simulink model "UNIFIER_dyn3DOF"  (R2023b)
settings: Solver=VariableStepAuto  StartTime=0.0  StopTime=0  RelTol=1e-3
InitFcn:
  | UNIFIER_LOAD
values from neighbouring files (symbols this model uses):
  b = 20.11467    [UNIFIER_LOAD.m]    (also in UNIFIER_LOAD.mat; UNIFIER_LOAD_ROM.m; UNIFIER_LOAD_ROM.mat)
  c = 1.43676    [UNIFIER_LOAD.m]    (also in UNIFIER_LOAD.mat; UNIFIER_LOAD_ROM.m; UNIFIER_LOAD_ROM.mat)
  dp_DEP =     [UNIFIER_LOAD.mat]    (also in UNIFIER_LOAD_ROM.mat)
  dp_FUSE_FIN =     [UNIFIER_LOAD.mat]
  dp_HTU =     [UNIFIER_LOAD.mat]    (also in UNIFIER_LOAD_ROM.mat)
  dp_VTAIL =     [UNIFIER_LOAD.mat]
  dp_VTAIL_INDUCED =     [UNIFIER_LOAD.mat]
  dp_WING_root =     [UNIFIER_LOAD.mat]
  dp_WING_tip =     [UNIFIER_LOAD.mat]
  I = [23600,     -0,  -1740 ... (first row only)    [UNIFIER_LOAD.m]    (also in UNIFIER_LOAD.mat = [23600  0  -1740; 0  89800  0; -1740  0  102000]; UNIFIER_LOAD_ROM.m = [23600,     -0,   -1740; UNIFIER_LOAD_ROM.mat = [23600  0  -1740; 0  89800  0; -1740  0  102000])
  m = 7057    [UNIFIER_LOAD.m]    (also in UNIFIER_LOAD.mat; UNIFIER_LOAD_ROM.m; UNIFIER_LOAD_ROM.mat)
  S = 29.98388    [UNIFIER_LOAD.m]    (also in UNIFIER_LOAD.mat; UNIFIER_LOAD_ROM.m; UNIFIER_LOAD_ROM.mat)
  vtail_nodes = [dp_VTAIL.Xs_LE;     dp_VTAIL.Ys_LE;     dp_VTAIL.Zs_LE]    [UNIFIER_LOAD.m]    (also in UNIFIER_LOAD.mat = [-16.4894695282 -2.83441376686 -2.73765826225 -16.1370849609)
  wing_nodes = [fliplr(dp_WING_tip.LE_Xs),fliplr(dp_WING_root.LE_Xs),dp_WING_root.LE_Xs,dp_WING_tip.LE_Xs;     fliplr(-dp_WING_tip.LE_Ys),fliplr(-dp_WING_root.LE_Ys),dp_WING_root.LE_Ys,dp_WING_tip.LE_Ys;     fliplr(dp_WING_tip.LE_Zs),fliplr(dp_WING_root.LE_Zs),dp_WING_root.LE_Zs,dp_WING_tip.LE_Zs]    [UNIFIER_LOAD.m]    (also in UNIFIER_LOAD.mat = [-7.70795631409 -9.67500019073 -0.98178178072 -7.66801691055)
  xyz_cg = [-8.09,0,-0.2]    [UNIFIER_LOAD.m]    (also in UNIFIER_LOAD.mat = [-8.09 0 -0.2]; UNIFIER_LOAD_ROM.m; UNIFIER_LOAD_ROM.mat = [-8.09 0 -0.2])
  xyz_DEP = [ -6.9629998	-6.9210000	-6.8660002	-6.8099999	-6.7540002	-6.6999998	-6.6999998	-6.7540002	-6.8099999	-6.8660002	-6.9210000	-6.9629998 ... (first row only)    [UNIFIER_LOAD.m]    (also in UNIFIER_LOAD.mat = [-6.9629998 -10.05 -0.90899998 -6.921 -8.4499998 -0.792 -6.8; UNIFIER_LOAD_ROM.m; UNIFIER_LOAD_ROM.mat = [-6.9629998 -10.05 -0.90899998 -6.921 -8.4499998 -0.792 -6.8)
undefined symbols (not defined in the file or in its folder): OBM, unifier_obm
libraries: sharedutil x7, aerolibtransform2 x4, sharedtransform x2, aerolibatmos2 x1, matrix_library x1, shared6dofsys x1, shared6dof x1, simulink x1
(part 2 of 3)

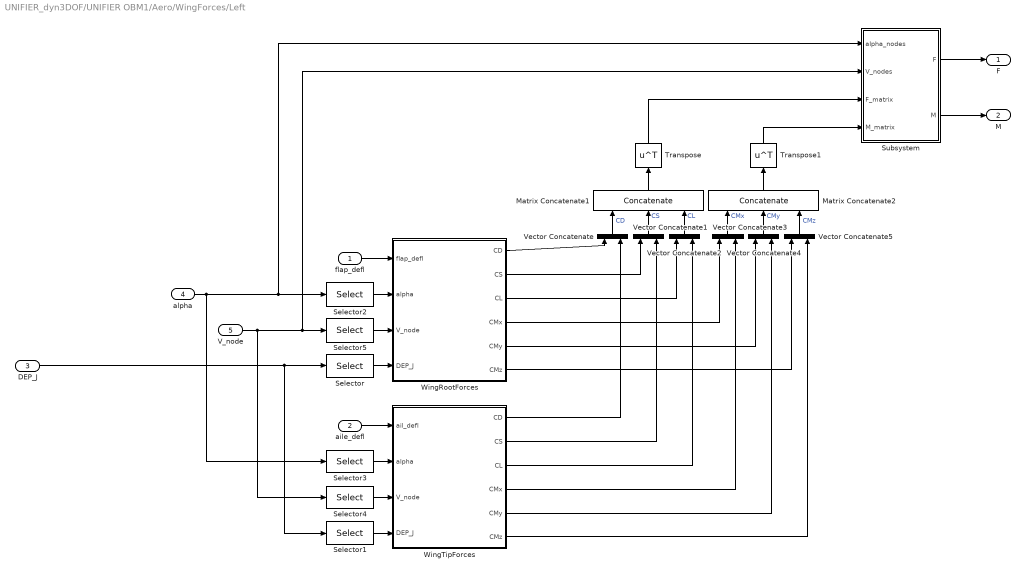
== system UNIFIER_dyn3DOF/UNIFIER OBM1/Aero/WingForces/Left ==
  flap_defl : Inport
  aile_defl : Inport  Port=2
  DEP_J : Inport  Port=3  PortDimensions=6
  alpha : Inport  Port=4  PortDimensions=7
  V_node : Inport  Port=5  PortDimensions=7
  Matrix Concatenate1 : Concatenate  NumInputs=3  Mode=Multidimensional array  ConcatenateDimension=2
  Matrix Concatenate2 : Concatenate  NumInputs=3  Mode=Multidimensional array  ConcatenateDimension=2
  Selector : Selector  InputPortWidth=6  IndexOptions=Index vector (dialog)  Indices=[1,2,3,4,5]  OutputSizes=1
  Selector1 : Selector  InputPortWidth=6  IndexOptions=Index vector (dialog)  Indices=[5,6]  OutputSizes=1
  Selector2 : Selector  InputPortWidth=7  IndexOptions=Index vector (dialog)  Indices=[1,2,3,4,5]  OutputSizes=1
  Selector3 : Selector  InputPortWidth=7  IndexOptions=Index vector (dialog)  Indices=[6,7]  OutputSizes=1
  Selector4 : Selector  InputPortWidth=7  IndexOptions=Index vector (dialog)  Indices=[6,7]  OutputSizes=1
  Selector5 : Selector  InputPortWidth=7  IndexOptions=Index vector (dialog)  Indices=[1,2,3,4,5]  OutputSizes=1
  Subsystem : Subsystem
  Transpose : Math  Operator=transpose
  Transpose1 : Math  Operator=transpose
  Vector Concatenate{,1..5} (6 alike) : Concatenate
  WingRootForces : Subsystem
  WingTipForces : Subsystem
  F : Outport
  M : Outport  Port=2
  wires:
  Subsystem/2(M) -> M/1
  Subsystem/1(F) -> F/1
  Transpose1/1 -> Subsystem/4(M_matrix)
  Transpose/1 -> Subsystem/3(F_matrix)
  Matrix Concatenate2/1 -> Transpose1/1
  Vector Concatenate5/1 -> Matrix Concatenate2/3  "CMz"
  Vector Concatenate4/1 -> Matrix Concatenate2/2  "CMy"
  Vector Concatenate3/1 -> Matrix Concatenate2/1  "CMx"
  Vector Concatenate2/1 -> Matrix Concatenate1/3  "CL"
  Vector Concatenate/1 -> Matrix Concatenate1/1  "CD"
  Matrix Concatenate1/1 -> Transpose/1
  Vector Concatenate1/1 -> Matrix Concatenate1/2  "CS"
  WingRootForces/5(CMy) -> Vector Concatenate4/1
  WingRootForces/4(CMx) -> Vector Concatenate3/1
  WingRootForces/3(CL) -> Vector Concatenate2/1
  WingRootForces/2(CS) -> Vector Concatenate1/1
  Selector5/1 -> WingRootForces/3(V_node)
  Selector4/1 -> WingTipForces/3(V_node)
  Selector3/1 -> WingTipForces/2(alpha)
  Selector2/1 -> WingRootForces/2(alpha)
  aile_defl/1 -> WingTipForces/1(ail_defl)
  WingTipForces/4(CMx) -> Vector Concatenate3/2
  WingTipForces/5(CMy) -> Vector Concatenate4/2
  WingTipForces/3(CL) -> Vector Concatenate2/2
  WingTipForces/2(CS) -> Vector Concatenate1/2
  WingTipForces/6(CMz) -> Vector Concatenate5/2
  WingTipForces/1(CD) -> Vector Concatenate/2
  WingRootForces/6(CMz) -> Vector Concatenate5/1
  Selector1/1 -> WingTipForces/4(DEP_J)
  WingRootForces/1(CD) -> Vector Concatenate/1
  V_node/1 -> Selector5/1, Subsystem/2(V_nodes), Selector4/1
  Selector/1 -> WingRootForces/4(DEP_J)
  DEP_J/1 -> Selector/1, Selector1/1
  alpha/1 -> Selector3/1, Selector2/1, Subsystem/1(alpha_nodes)
  flap_defl/1 -> WingRootForces/1(flap_defl)

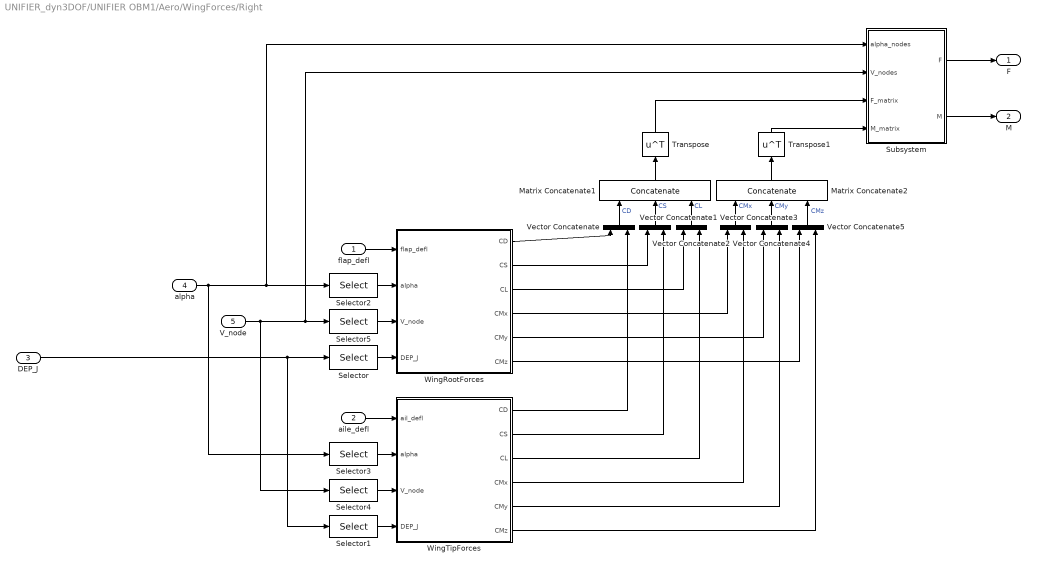
== system UNIFIER_dyn3DOF/UNIFIER OBM1/Aero/WingForces/Right ==
  flap_defl : Inport
  aile_defl : Inport  Port=2
  DEP_J : Inport  Port=3  PortDimensions=6
  alpha : Inport  Port=4  PortDimensions=7
  V_node : Inport  Port=5  PortDimensions=7
  Matrix Concatenate1 : Concatenate  NumInputs=3  Mode=Multidimensional array  ConcatenateDimension=2
  Matrix Concatenate2 : Concatenate  NumInputs=3  Mode=Multidimensional array  ConcatenateDimension=2
  Selector : Selector  InputPortWidth=6  IndexOptions=Index vector (dialog)  Indices=[1,2,3,4,5]  OutputSizes=1
  Selector1 : Selector  InputPortWidth=6  IndexOptions=Index vector (dialog)  Indices=[5,6]  OutputSizes=1
  Selector2 : Selector  InputPortWidth=7  IndexOptions=Index vector (dialog)  Indices=[1,2,3,4,5]  OutputSizes=1
  Selector3 : Selector  InputPortWidth=7  IndexOptions=Index vector (dialog)  Indices=[6,7]  OutputSizes=1
  Selector4 : Selector  InputPortWidth=7  IndexOptions=Index vector (dialog)  Indices=[6,7]  OutputSizes=1
  Selector5 : Selector  InputPortWidth=7  IndexOptions=Index vector (dialog)  Indices=[1,2,3,4,5]  OutputSizes=1
  Subsystem : Subsystem
  Transpose : Math  Operator=transpose
  Transpose1 : Math  Operator=transpose
  Vector Concatenate{,1..5} (6 alike) : Concatenate
  WingRootForces : Subsystem
  WingTipForces : Subsystem
  F : Outport
  M : Outport  Port=2
  wires:
  Subsystem/2(M) -> M/1
  Subsystem/1(F) -> F/1
  Transpose1/1 -> Subsystem/4(M_matrix)
  Transpose/1 -> Subsystem/3(F_matrix)
  Matrix Concatenate2/1 -> Transpose1/1
  Vector Concatenate5/1 -> Matrix Concatenate2/3  "CMz"
  Vector Concatenate4/1 -> Matrix Concatenate2/2  "CMy"
  Vector Concatenate3/1 -> Matrix Concatenate2/1  "CMx"
  Vector Concatenate2/1 -> Matrix Concatenate1/3  "CL"
  Vector Concatenate/1 -> Matrix Concatenate1/1  "CD"
  Matrix Concatenate1/1 -> Transpose/1
  Vector Concatenate1/1 -> Matrix Concatenate1/2  "CS"
  WingRootForces/5(CMy) -> Vector Concatenate4/1
  WingRootForces/4(CMx) -> Vector Concatenate3/1
  WingRootForces/3(CL) -> Vector Concatenate2/1
  WingRootForces/2(CS) -> Vector Concatenate1/1
  Selector5/1 -> WingRootForces/3(V_node)
  Selector4/1 -> WingTipForces/3(V_node)
  Selector3/1 -> WingTipForces/2(alpha)
  Selector2/1 -> WingRootForces/2(alpha)
  aile_defl/1 -> WingTipForces/1(ail_defl)
  WingTipForces/4(CMx) -> Vector Concatenate3/2
  WingTipForces/5(CMy) -> Vector Concatenate4/2
  WingTipForces/3(CL) -> Vector Concatenate2/2
  WingTipForces/2(CS) -> Vector Concatenate1/2
  WingTipForces/6(CMz) -> Vector Concatenate5/2
  WingTipForces/1(CD) -> Vector Concatenate/2
  WingRootForces/6(CMz) -> Vector Concatenate5/1
  Selector1/1 -> WingTipForces/4(DEP_J)
  WingRootForces/1(CD) -> Vector Concatenate/1
  V_node/1 -> Selector5/1, Subsystem/2(V_nodes), Selector4/1
  Selector/1 -> WingRootForces/4(DEP_J)
  DEP_J/1 -> Selector/1, Selector1/1
  alpha/1 -> Selector3/1, Selector2/1, Subsystem/1(alpha_nodes)
  flap_defl/1 -> WingRootForces/1(flap_defl)

== system UNIFIER_dyn3DOF/UNIFIER OBM1/Aero/WingForces/Subsystem ==
  DEP_J : Inport
  alpha_nodes : Inport  Port=2
  V_nodes : Inport  Port=3
  Demux1 : Demux  Outputs=2
  Demux2 : Demux  Outputs=2
  Demux3 : Demux  Outputs=2
  Selector : Selector  InputPortWidth=6  IndexOptions=Index vector (dialog)  Indices=[6,5,4,3,2,1]  OutputSizes=1
  Selector1 : Selector  InputPortWidth=7  IndexOptions=Index vector (dialog)  Indices=[7,6,5,4,3,2,1]  OutputSizes=1
  Selector2 : Selector  InputPortWidth=7  IndexOptions=Index vector (dialog)  Indices=[7,6,5,4,3,2,1]  OutputSizes=1
  DEP_J_Left : Outport  PortDimensions=6
  alpha_nodes_Left : Outport  Port=2  PortDimensions=7
  V_nodes_Left : Outport  Port=3  PortDimensions=7
  DEP_J_Right : Outport  Port=4  PortDimensions=6
  alpha_nodes_Right : Outport  Port=5  PortDimensions=7
  V_nodes_Right : Outport  Port=6  PortDimensions=7
  wires:
  Demux3/2 -> V_nodes_Right/1
  V_nodes/1 -> Demux3/1
  Selector2/1 -> V_nodes_Left/1
  Demux3/1 -> Selector2/1
  Demux1/1 -> Selector1/1
  Demux1/2 -> alpha_nodes_Right/1
  alpha_nodes/1 -> Demux1/1
  Selector1/1 -> alpha_nodes_Left/1
  Selector/1 -> DEP_J_Left/1
  DEP_J/1 -> Demux2/1
  Demux2/1 -> Selector/1
  Demux2/2 -> DEP_J_Right/1

== system UNIFIER_dyn3DOF/UNIFIER OBM1/EOMandEnviroment/EOM/Subsystem ==
  p q r : Inport
  phi theta psi : Inport  Port=2
  Mux1 : Mux  Inputs=[3 3 3]
  Mux2 : Mux  Inputs=3
  phidot : Fcn  Expr=u[1]+(u[2]*u[4]+u[3]*u[7])*(u[5]/u[8])
  psidot : Fcn  Expr=(u[2]*u[4]+u[3]*u[7])/u[8]
  sincos : Trigonometry  Operator=sincos
  thetadot : Fcn  Expr=u[2]*u[7]-u[3]*u[4]
  phidot thetadot psidot : Outport  InitialOutput=0  VectorParamsAs1DForOutWhenUnconnected=off
  wires:
  sincos/2 -> Mux1/3
  phi theta psi/1 -> sincos/1
  phidot/1 -> Mux2/1
  Mux2/1 -> phidot thetadot psidot/1
  p q r/1 -> Mux1/1
  thetadot/1 -> Mux2/2
  psidot/1 -> Mux2/3
  sincos/1 -> Mux1/2
  Mux1/1 -> thetadot/1, phidot/1, psidot/1

== system UNIFIER_dyn3DOF/UNIFIER OBM1/Subsystems/DEP1/AngularVelocityComponent ==
  r : Inport
  Constant : Constant  Value=xyz_DEP
  Constant4 : Constant  Value=xyz_cg
  Gain : Gain  Gain=ones(1,12)
  Product : Product
  Reshape : Reshape
  Reshape3 : Reshape
  Selector1 : Selector  NumberOfDimensions=2  InputPortWidth=6  IndexOptions=Index vector (dialog),Select all  Indices=2,1  OutputSizes=1,1
  Selector3 : Selector  InputPortWidth=3  IndexOptions=Index vector (dialog)  Indices=2  OutputSizes=1
  Sum1 : Sum  Inputs=|+-
  u_induced : Outport
  wires:
  Product/1 -> u_induced/1
  Reshape/1 -> Sum1/2
  Constant/1 -> Selector1/1
  r/1 -> Product/1
  Reshape3/1 -> Sum1/1
  Gain/1 -> Reshape3/1
  Selector3/1 -> Gain/1
  Sum1/1 -> Product/2
  Constant4/1 -> Selector3/1
  Selector1/1 -> Reshape/1

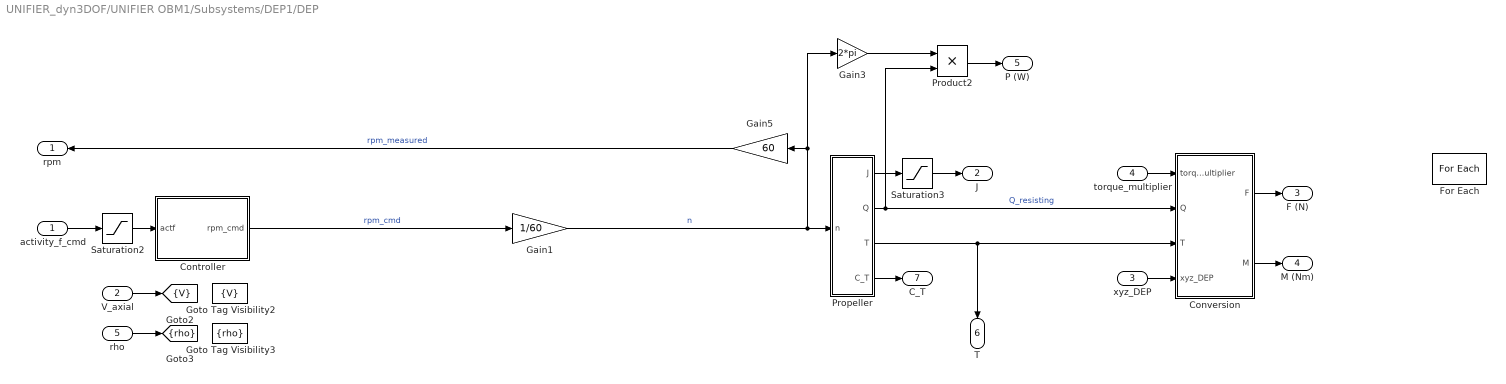
== system UNIFIER_dyn3DOF/UNIFIER OBM1/Subsystems/DEP1/DEP ==
  activity_f_cmd : Inport  Partition=on  PartitionDimension=1  PartitionWidth=1  PartitionOffset=0
  V_axial : Inport  Port=2  Partition=on  PartitionDimension=1  PartitionWidth=1  PartitionOffset=0
  xyz_DEP : Inport  Port=3  Partition=on  PartitionDimension=2  PartitionWidth=1  PartitionOffset=0
  torque_multiplier : Inport  Port=4  Partition=on  PartitionDimension=1  PartitionWidth=1  PartitionOffset=0
  rho : Inport  Port=5
  Controller : Subsystem
  Conversion : Subsystem
  For Each : ForEach  DisableCoverage=on  SpecifiedNumIters=12
  Gain1 : Gain  Gain=1/60
  Gain3 : Gain  Gain=2*pi
  Gain5 : Gain  Gain=60
  Goto Tag Visibility2 : GotoTagVisibility  GotoTag=V
  Goto Tag Visibility3 : GotoTagVisibility  GotoTag=rho
  Product2 : Product
  Propeller : Subsystem
  Saturation2 : Saturate  UpperLimit=1  LowerLimit=0
  Saturation3 : Saturate  UpperLimit=5  LowerLimit=0.2
  rpm : Outport  ConcatenationDimension=1
  J : Outport  Port=2  ConcatenationDimension=1
  F (N) : Outport  Port=3  ConcatenationDimension=2
  M (Nm) : Outport  Port=4  ConcatenationDimension=2
  P (W) : Outport  Port=5  ConcatenationDimension=1
  T : Outport  Port=6  ConcatenationDimension=1
  C_T : Outport  Port=7  ConcatenationDimension=1
  tag scope: V=scoped, rho=scoped
  wires:
  Controller/1(rpm_cmd) -> Gain1/1  "rpm_cmd"
  Saturation2/1 -> Controller/1(actf)
  Propeller/2(Q) -> Conversion/2(Q), Product2/2  "Q_resisting"
  rho/1 -> [rho]
  Propeller/3(T) -> Conversion/3(T), T/1
  Gain5/1 -> rpm/1  "rpm_measured"
  torque_multiplier/1 -> Conversion/1(torque_multiplier)
  Product2/1 -> P (W)/1
  V_axial/1 -> [V]
  Gain1/1 -> Propeller/1(n), Gain5/1, Gain3/1  "n"
  xyz_DEP/1 -> Conversion/4(xyz_DEP)
  Gain3/1 -> Product2/1
  Propeller/1(J) -> Saturation3/1
  activity_f_cmd/1 -> Saturation2/1
  Propeller/4(C_T) -> C_T/1
  Saturation3/1 -> J/1
  Conversion/2(M) -> M (Nm)/1
  Conversion/1(F) -> F (N)/1

== system UNIFIER_dyn3DOF/UNIFIER OBM1/Subsystems/HTU/PropAndMotor ==
  Vrw_mag_eas : Inport
  T_cmd (N) : Inport  Port=2
  1-D Lookup Table : Lookup_n-D  NumberOfTableDimensions=1  BreakpointsForDimension1=dp_HTU.limits.V_low_lim  IndexSearchMethod=Linear search  BeginIndexSearchUsingPreviousIndexResult=on  Table=dp_HTU.limits.T_low_lim  InternalRulePriority=Speed  RndMeth=Simplest
  1-D Lookup Table1 : Lookup_n-D  NumberOfTableDimensions=1  BreakpointsForDimension1=dp_HTU.limits.V_up_lim  IndexSearchMethod=Linear search  BeginIndexSearchUsingPreviousIndexResult=on  Table=dp_HTU.limits.T_up_lim  InternalRulePriority=Speed  RndMeth=Simplest
  P lookup : Lookup_n-D  BreakpointsForDimension1=dp_HTU.V_vec  BreakpointsForDimension2=dp_HTU.T_vec  IndexSearchMethod=Linear search  BeginIndexSearchUsingPreviousIndexResult=on  Table=dp_HTU.P_grid  InternalRulePriority=Speed  RndMeth=Simplest
      settings: InputPortMap=u0,u1
  Saturation Dynamic : simulink/Discontinuities/Saturation Dynamic  OutMin=[]  OutMax=[]  OutDataTypeStr=Inherit: Same as second input  OutDataType=fixdt(1, 16)  OutScaling=2^-10  DoSatur=off
  P (kW) : Outport
  T (N) : Outport  Port=2
  wires:
  Saturation Dynamic/1 -> P lookup/2, T (N)/1
  T_cmd (N)/1 -> Saturation Dynamic/2
  1-D Lookup Table/1 -> Saturation Dynamic/3
  1-D Lookup Table1/1 -> Saturation Dynamic/1
  P lookup/1 -> P (kW)/1
  Vrw_mag_eas/1 -> 1-D Lookup Table1/1, 1-D Lookup Table/1, P lookup/1

== system UNIFIER_dyn3DOF/UNIFIER OBM1/Aero/FinFuselageForces/Subsystem1/Subsystem ==
  beta : Inport
  alpha : Inport  Port=2
  Prelookup : PreLookup  BreakpointsData=dp_FUSE_FIN.beta  IndexSearchMethod=Linear search  BeginIndexSearchUsingPreviousIndexResult=on  ExtrapMethod=Linear
  Prelookup1 : PreLookup  BreakpointsData=dp_FUSE_FIN.aoa  IndexSearchMethod=Linear search  BeginIndexSearchUsingPreviousIndexResult=on  ExtrapMethod=Linear
  Out1 : Outport
  Out2 : Outport  Port=2
  Out3 : Outport  Port=3
  Out4 : Outport  Port=4
  wires:
  Prelookup/2 -> Out2/1
  Prelookup1/2 -> Out4/1
  Prelookup1/1 -> Out3/1
  beta/1 -> Prelookup/1
  alpha/1 -> Prelookup1/1
  Prelookup/1 -> Out1/1

== system UNIFIER_dyn3DOF/UNIFIER OBM1/Aero/VtailForces/Subsystem/CrossProduct1 ==
  r : Inport  Partition=on  PartitionDimension=2  PartitionWidth=1  PartitionOffset=0
  F : Inport  Port=2  Partition=on  PartitionDimension=2  PartitionWidth=1  PartitionOffset=0
  3x3 Cross Product : sharedutil/3x3 Cross Product  aMode=aMode
  CG : Constant  Value=xyz_cg
  Cast : DataTypeConversion  OutDataTypeStr=single  SaturateOnIntegerOverflow=off  RndMeth=Floor
  For Each : ForEach  DisableCoverage=on  SpecifiedNumIters=16
  Minus : Sum  Inputs=+-
  M : Outport  ConcatenationDimension=2
  wires:
  Cast/1 -> Minus/2
  Minus/1 -> 3x3 Cross Product/1
  CG/1 -> Cast/1
  3x3 Cross Product/1 -> M/1
  r/1 -> Minus/1
  F/1 -> 3x3 Cross Product/2

== system UNIFIER_dyn3DOF/UNIFIER OBM1/Aero/VtailForces/VtailForces/WingRootPreLookup ==
  rude_defl_nodes : Inport
  alpha_nodes : Inport  Port=2
  beta_nodes : Inport  Port=3
  Constant8 : Constant  Value=0:15
  Prelookup : PreLookup  BreakpointsData=dp_VTAIL.rude_defl  IndexSearchMethod=Linear search  BeginIndexSearchUsingPreviousIndexResult=on  ExtrapMethod=Linear
  Prelookup1 : PreLookup  BreakpointsData=dp_VTAIL.alphas  IndexSearchMethod=Linear search  BeginIndexSearchUsingPreviousIndexResult=on  ExtrapMethod=Linear
  Prelookup2 : PreLookup  BreakpointsData=dp_VTAIL.betas  IndexSearchMethod=Linear search  BeginIndexSearchUsingPreviousIndexResult=on  ExtrapMethod=Linear
  Out1 : Outport
  Out2 : Outport  Port=2
  Out3 : Outport  Port=3
  Out4 : Outport  Port=4
  Out6 : Outport  Port=5
  Out7 : Outport  Port=6
  Out5 : Outport  Port=7
  wires:
  Prelookup2/2 -> Out7/1
  Prelookup2/1 -> Out6/1
  beta_nodes/1 -> Prelookup2/1
  rude_defl_nodes/1 -> Prelookup/1
  Prelookup1/1 -> Out3/1
  alpha_nodes/1 -> Prelookup1/1
  Prelookup/2 -> Out2/1
  Prelookup1/2 -> Out4/1
  Constant8/1 -> Out5/1
  Prelookup/1 -> Out1/1

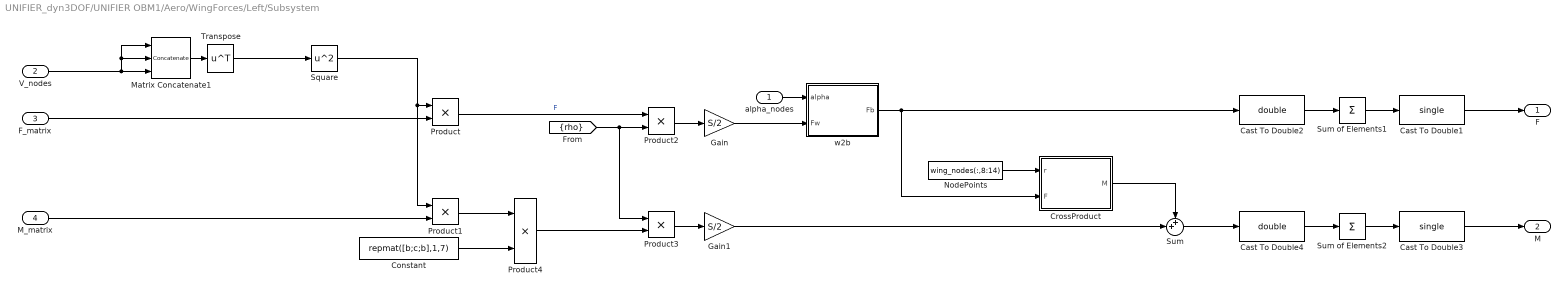
== system UNIFIER_dyn3DOF/UNIFIER OBM1/Aero/WingForces/Left/Subsystem ==
  alpha_nodes : Inport
  V_nodes : Inport  Port=2
  F_matrix : Inport  Port=3
  M_matrix : Inport  Port=4
  Cast To Double1 : DataTypeConversion  OutDataTypeStr=single  SaturateOnIntegerOverflow=off  RndMeth=Floor
  Cast To Double2 : DataTypeConversion  OutDataTypeStr=double  SaturateOnIntegerOverflow=off  RndMeth=Floor
  Cast To Double3 : DataTypeConversion  OutDataTypeStr=single  SaturateOnIntegerOverflow=off  RndMeth=Floor
  Cast To Double4 : DataTypeConversion  OutDataTypeStr=double  SaturateOnIntegerOverflow=off  RndMeth=Floor
  Constant : Constant  Value=repmat([b;c;b],1,7)
  CrossProduct : Subsystem  TreatAsAtomicUnit=on
  Gain : Gain  Gain=S/2
  Gain1 : Gain  Gain=S/2
  Matrix Concatenate1 : Concatenate  NumInputs=3  Mode=Multidimensional array  ConcatenateDimension=2
  NodePoints : Constant  Value=wing_nodes(:,8:14)
  Product{,1..4} (5 alike) : Product
  Square : Math  Operator=square
  Sum : Sum  Inputs=++|
  Sum of Elements1 : Sum  Inputs=+  CollapseMode=Specified dimension  CollapseDim=2
  Sum of Elements2 : Sum  Inputs=+  CollapseMode=Specified dimension  CollapseDim=2
  Transpose : Math  Operator=transpose
  w2b : Subsystem  TreatAsAtomicUnit=on
  F : Outport
  M : Outport  Port=2
  wires:
  Cast To Double3/1 -> M/1
  Sum/1 -> Cast To Double4/1
  Cast To Double4/1 -> Sum of Elements2/1
  Sum of Elements2/1 -> Cast To Double3/1
  Sum of Elements1/1 -> Cast To Double1/1
  Cast To Double2/1 -> Sum of Elements1/1
  alpha_nodes/1 -> w2b/1(alpha)
  Gain/1 -> w2b/2(Fw)
  Cast To Double1/1 -> F/1
  CrossProduct/1(M) -> Sum/1
  NodePoints/1 -> CrossProduct/1(r)
  w2b/1(Fb) -> CrossProduct/2(F), Cast To Double2/1
  Square/1 -> Product/1, Product1/1
  Matrix Concatenate1/1 -> Transpose/1
  Transpose/1 -> Square/1
  V_nodes/1 -> Matrix Concatenate1/3, Matrix Concatenate1/2, Matrix Concatenate1/1
  Product/1 -> Product2/1  "F"
  Gain1/1 -> Sum/2
  Product1/1 -> Product4/1
  M_matrix/1 -> Product1/2
  Product4/1 -> Product3/2
  Constant/1 -> Product4/2
  Product3/1 -> Gain1/1
  [rho] -> Product2/2, Product3/1
  F_matrix/1 -> Product/2
  Product2/1 -> Gain/1

== system UNIFIER_dyn3DOF/UNIFIER OBM1/Aero/WingForces/Left/WingRootForces ==
  flap_defl : Inport
  alpha : Inport  Port=2
  V_node : Inport  Port=3
  DEP_J : Inport  Port=4
  Interpolation Using Prelookup1 : Interpolation_n-D  NumberOfTableDimensions=5  Table=dp_WING_root.CD  ExtrapMethod=Clip  ValidIndexMayReachLast=on  NumSelectionDims=1  InternalRulePriority=Speed  TableDataTypeStr=Inherit: Inherit from 'Table data'
      settings: InputPortMap=u0,u1,u2,u3,u4,u5,u6,u7,u8
  Interpolation Using Prelookup2 : Interpolation_n-D  NumberOfTableDimensions=5  Table=dp_WING_root.CS  ExtrapMethod=Clip  ValidIndexMayReachLast=on  NumSelectionDims=1  InternalRulePriority=Speed  TableDataTypeStr=Inherit: Inherit from 'Table data'
      settings: InputPortMap=u0,u1,u2,u3,u4,u5,u6,u7,u8
  Interpolation Using Prelookup3 : Interpolation_n-D  NumberOfTableDimensions=5  Table=dp_WING_root.CL  ExtrapMethod=Clip  ValidIndexMayReachLast=on  NumSelectionDims=1  InternalRulePriority=Speed  TableDataTypeStr=Inherit: Inherit from 'Table data'
      settings: InputPortMap=u0,u1,u2,u3,u4,u5,u6,u7,u8
  Interpolation Using Prelookup4 : Interpolation_n-D  NumberOfTableDimensions=5  Table=dp_WING_root.CMx  ExtrapMethod=Clip  ValidIndexMayReachLast=on  NumSelectionDims=1  InternalRulePriority=Speed  TableDataTypeStr=Inherit: Inherit from 'Table data'
      settings: InputPortMap=u0,u1,u2,u3,u4,u5,u6,u7,u8
  Interpolation Using Prelookup5 : Interpolation_n-D  NumberOfTableDimensions=5  Table=dp_WING_root.CMy  ExtrapMethod=Clip  ValidIndexMayReachLast=on  NumSelectionDims=1  InternalRulePriority=Speed  TableDataTypeStr=Inherit: Inherit from 'Table data'
      settings: InputPortMap=u0,u1,u2,u3,u4,u5,u6,u7,u8
  Interpolation Using Prelookup6 : Interpolation_n-D  NumberOfTableDimensions=5  Table=dp_WING_root.CMz  ExtrapMethod=Clip  ValidIndexMayReachLast=on  NumSelectionDims=1  InternalRulePriority=Speed  TableDataTypeStr=Inherit: Inherit from 'Table data'
      settings: InputPortMap=u0,u1,u2,u3,u4,u5,u6,u7,u8
  WingRootPreLookup : Subsystem
  CD : Outport
  CS : Outport  Port=2
  CL : Outport  Port=3
  CMx : Outport  Port=4
  CMy : Outport  Port=5
  CMz : Outport  Port=6
  wires:
  Interpolation Using Prelookup6/1 -> CMz/1
  Interpolation Using Prelookup5/1 -> CMy/1
  Interpolation Using Prelookup4/1 -> CMx/1
  Interpolation Using Prelookup3/1 -> CL/1
  Interpolation Using Prelookup2/1 -> CS/1
  alpha/1 -> WingRootPreLookup/2(alpha)
  V_node/1 -> WingRootPreLookup/3(V_node)
  DEP_J/1 -> WingRootPreLookup/4(DEP_J)
  WingRootPreLookup/2(Out2) -> Interpolation Using Prelookup1/2, Interpolation Using Prelookup2/2, Interpolation Using Prelookup3/2, Interpolation Using Prelookup4/2, Interpolation Using Prelookup5/2, Interpolation Using Prelookup6/2
  WingRootPreLookup/6(Out7) -> Interpolation Using Prelookup1/6, Interpolation Using Prelookup2/6, Interpolation Using Prelookup3/6, Interpolation Using Prelookup4/6, Interpolation Using Prelookup5/6, Interpolation Using Prelookup6/6
  Interpolation Using Prelookup1/1 -> CD/1
  WingRootPreLookup/5(Out6) -> Interpolation Using Prelookup2/5, Interpolation Using Prelookup3/5, Interpolation Using Prelookup4/5, Interpolation Using Prelookup5/5, Interpolation Using Prelookup6/5, Interpolation Using Prelookup1/5
  WingRootPreLookup/4(Out4) -> Interpolation Using Prelookup1/4, Interpolation Using Prelookup2/4, Interpolation Using Prelookup3/4, Interpolation Using Prelookup4/4, Interpolation Using Prelookup5/4, Interpolation Using Prelookup6/4
  flap_defl/1 -> WingRootPreLookup/1(flap_defl)
  WingRootPreLookup/7(Out8) -> Interpolation Using Prelookup2/7, Interpolation Using Prelookup3/7, Interpolation Using Prelookup4/7, Interpolation Using Prelookup6/7, Interpolation Using Prelookup5/7, Interpolation Using Prelookup1/7
  WingRootPreLookup/1(Out1) -> Interpolation Using Prelookup1/1, Interpolation Using Prelookup2/1, Interpolation Using Prelookup3/1, Interpolation Using Prelookup4/1, Interpolation Using Prelookup5/1, Interpolation Using Prelookup6/1
  WingRootPreLookup/8(Out9) -> Interpolation Using Prelookup1/8, Interpolation Using Prelookup2/8, Interpolation Using Prelookup3/8, Interpolation Using Prelookup4/8, Interpolation Using Prelookup5/8, Interpolation Using Prelookup6/8
  WingRootPreLookup/3(Out3) -> Interpolation Using Prelookup1/3, Interpolation Using Prelookup2/3, Interpolation Using Prelookup3/3, Interpolation Using Prelookup4/3, Interpolation Using Prelookup5/3, Interpolation Using Prelookup6/3
  WingRootPreLookup/9(Out5) -> Interpolation Using Prelookup1/9, Interpolation Using Prelookup2/9, Interpolation Using Prelookup3/9, Interpolation Using Prelookup4/9, Interpolation Using Prelookup5/9, Interpolation Using Prelookup6/9

== system UNIFIER_dyn3DOF/UNIFIER OBM1/Aero/WingForces/Left/WingTipForces ==
  ail_defl : Inport
  alpha : Inport  Port=2
  V_node : Inport  Port=3
  DEP_J : Inport  Port=4
  Interpolation Using Prelookup1 : Interpolation_n-D  NumberOfTableDimensions=5  Table=dp_WING_tip.CD  ExtrapMethod=Clip  ValidIndexMayReachLast=on  NumSelectionDims=1  InternalRulePriority=Speed  TableDataTypeStr=Inherit: Inherit from 'Table data'
      settings: InputPortMap=u0,u1,u2,u3,u4,u5,u6,u7,u8
  Interpolation Using Prelookup2 : Interpolation_n-D  NumberOfTableDimensions=5  Table=dp_WING_tip.CS  ExtrapMethod=Clip  ValidIndexMayReachLast=on  NumSelectionDims=1  InternalRulePriority=Speed  TableDataTypeStr=Inherit: Inherit from 'Table data'
      settings: InputPortMap=u0,u1,u2,u3,u4,u5,u6,u7,u8
  Interpolation Using Prelookup3 : Interpolation_n-D  NumberOfTableDimensions=5  Table=dp_WING_tip.CL  ExtrapMethod=Clip  ValidIndexMayReachLast=on  NumSelectionDims=1  InternalRulePriority=Speed  TableDataTypeStr=Inherit: Inherit from 'Table data'
      settings: InputPortMap=u0,u1,u2,u3,u4,u5,u6,u7,u8
  Interpolation Using Prelookup4 : Interpolation_n-D  NumberOfTableDimensions=5  Table=dp_WING_tip.CMx  ExtrapMethod=Clip  ValidIndexMayReachLast=on  NumSelectionDims=1  InternalRulePriority=Speed  TableDataTypeStr=Inherit: Inherit from 'Table data'
      settings: InputPortMap=u0,u1,u2,u3,u4,u5,u6,u7,u8
  Interpolation Using Prelookup5 : Interpolation_n-D  NumberOfTableDimensions=5  Table=dp_WING_tip.CMy  ExtrapMethod=Clip  ValidIndexMayReachLast=on  NumSelectionDims=1  InternalRulePriority=Speed  TableDataTypeStr=Inherit: Inherit from 'Table data'
      settings: InputPortMap=u0,u1,u2,u3,u4,u5,u6,u7,u8
  Interpolation Using Prelookup6 : Interpolation_n-D  NumberOfTableDimensions=5  Table=dp_WING_tip.CMz  ExtrapMethod=Clip  ValidIndexMayReachLast=on  NumSelectionDims=1  InternalRulePriority=Speed  TableDataTypeStr=Inherit: Inherit from 'Table data'
      settings: InputPortMap=u0,u1,u2,u3,u4,u5,u6,u7,u8
  WingRootPreLookup : Subsystem
  CD : Outport
  CS : Outport  Port=2
  CL : Outport  Port=3
  CMx : Outport  Port=4
  CMy : Outport  Port=5
  CMz : Outport  Port=6
  wires:
  Interpolation Using Prelookup6/1 -> CMz/1
  Interpolation Using Prelookup5/1 -> CMy/1
  Interpolation Using Prelookup4/1 -> CMx/1
  Interpolation Using Prelookup3/1 -> CL/1
  Interpolation Using Prelookup2/1 -> CS/1
  alpha/1 -> WingRootPreLookup/2(alpha)
  V_node/1 -> WingRootPreLookup/3(V_node)
  DEP_J/1 -> WingRootPreLookup/4(DEP_J)
  WingRootPreLookup/2(Out2) -> Interpolation Using Prelookup1/2, Interpolation Using Prelookup2/2, Interpolation Using Prelookup3/2, Interpolation Using Prelookup4/2, Interpolation Using Prelookup5/2, Interpolation Using Prelookup6/2
  WingRootPreLookup/6(Out7) -> Interpolation Using Prelookup1/6, Interpolation Using Prelookup2/6, Interpolation Using Prelookup3/6, Interpolation Using Prelookup4/6, Interpolation Using Prelookup5/6, Interpolation Using Prelookup6/6
  Interpolation Using Prelookup1/1 -> CD/1
  WingRootPreLookup/5(Out6) -> Interpolation Using Prelookup2/5, Interpolation Using Prelookup3/5, Interpolation Using Prelookup4/5, Interpolation Using Prelookup5/5, Interpolation Using Prelookup6/5, Interpolation Using Prelookup1/5
  WingRootPreLookup/4(Out4) -> Interpolation Using Prelookup1/4, Interpolation Using Prelookup2/4, Interpolation Using Prelookup3/4, Interpolation Using Prelookup4/4, Interpolation Using Prelookup5/4, Interpolation Using Prelookup6/4
  ail_defl/1 -> WingRootPreLookup/1(ail_defl)
  WingRootPreLookup/7(Out8) -> Interpolation Using Prelookup1/7, Interpolation Using Prelookup2/7, Interpolation Using Prelookup3/7, Interpolation Using Prelookup4/7, Interpolation Using Prelookup6/7, Interpolation Using Prelookup5/7
  WingRootPreLookup/1(Out1) -> Interpolation Using Prelookup1/1, Interpolation Using Prelookup2/1, Interpolation Using Prelookup3/1, Interpolation Using Prelookup4/1, Interpolation Using Prelookup5/1, Interpolation Using Prelookup6/1
  WingRootPreLookup/8(Out9) -> Interpolation Using Prelookup1/8, Interpolation Using Prelookup2/8, Interpolation Using Prelookup3/8, Interpolation Using Prelookup4/8, Interpolation Using Prelookup5/8, Interpolation Using Prelookup6/8
  WingRootPreLookup/3(Out3) -> Interpolation Using Prelookup1/3, Interpolation Using Prelookup2/3, Interpolation Using Prelookup3/3, Interpolation Using Prelookup4/3, Interpolation Using Prelookup5/3, Interpolation Using Prelookup6/3
  WingRootPreLookup/9(Out5) -> Interpolation Using Prelookup1/9, Interpolation Using Prelookup2/9, Interpolation Using Prelookup3/9, Interpolation Using Prelookup4/9, Interpolation Using Prelookup5/9, Interpolation Using Prelookup6/9

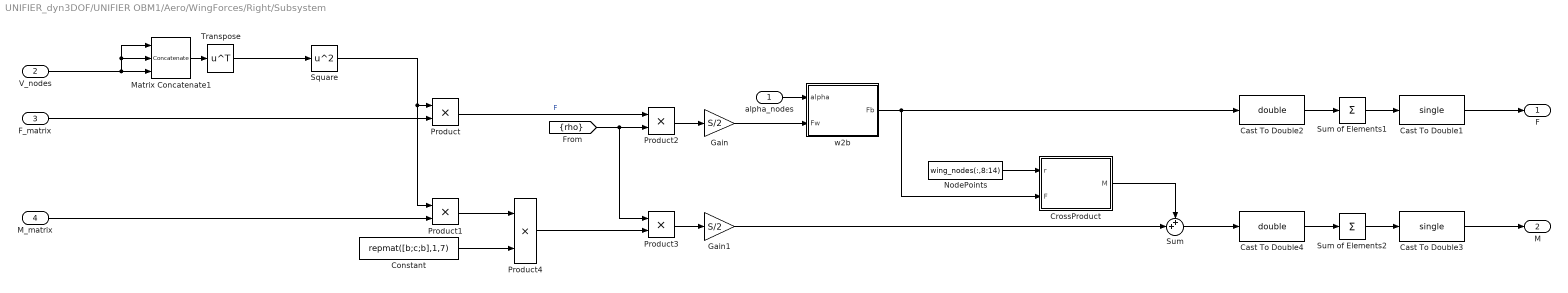
== system UNIFIER_dyn3DOF/UNIFIER OBM1/Aero/WingForces/Right/Subsystem ==
  alpha_nodes : Inport
  V_nodes : Inport  Port=2
  F_matrix : Inport  Port=3
  M_matrix : Inport  Port=4
  Cast To Double1 : DataTypeConversion  OutDataTypeStr=single  SaturateOnIntegerOverflow=off  RndMeth=Floor
  Cast To Double2 : DataTypeConversion  OutDataTypeStr=double  SaturateOnIntegerOverflow=off  RndMeth=Floor
  Cast To Double3 : DataTypeConversion  OutDataTypeStr=single  SaturateOnIntegerOverflow=off  RndMeth=Floor
  Cast To Double4 : DataTypeConversion  OutDataTypeStr=double  SaturateOnIntegerOverflow=off  RndMeth=Floor
  Constant : Constant  Value=repmat([b;c;b],1,7)
  CrossProduct : Subsystem  TreatAsAtomicUnit=on
  Gain : Gain  Gain=S/2
  Gain1 : Gain  Gain=S/2
  Matrix Concatenate1 : Concatenate  NumInputs=3  Mode=Multidimensional array  ConcatenateDimension=2
  NodePoints : Constant  Value=wing_nodes(:,8:14)
  Product{,1..4} (5 alike) : Product
  Square : Math  Operator=square
  Sum : Sum  Inputs=++|
  Sum of Elements1 : Sum  Inputs=+  CollapseMode=Specified dimension  CollapseDim=2
  Sum of Elements2 : Sum  Inputs=+  CollapseMode=Specified dimension  CollapseDim=2
  Transpose : Math  Operator=transpose
  w2b : Subsystem  TreatAsAtomicUnit=on
  F : Outport
  M : Outport  Port=2
  wires:
  Cast To Double3/1 -> M/1
  Sum/1 -> Cast To Double4/1
  Cast To Double4/1 -> Sum of Elements2/1
  Sum of Elements2/1 -> Cast To Double3/1
  Sum of Elements1/1 -> Cast To Double1/1
  Cast To Double2/1 -> Sum of Elements1/1
  alpha_nodes/1 -> w2b/1(alpha)
  Gain/1 -> w2b/2(Fw)
  Cast To Double1/1 -> F/1
  CrossProduct/1(M) -> Sum/1
  NodePoints/1 -> CrossProduct/1(r)
  w2b/1(Fb) -> CrossProduct/2(F), Cast To Double2/1
  Square/1 -> Product/1, Product1/1
  Matrix Concatenate1/1 -> Transpose/1
  Transpose/1 -> Square/1
  V_nodes/1 -> Matrix Concatenate1/3, Matrix Concatenate1/2, Matrix Concatenate1/1
  Product/1 -> Product2/1  "F"
  Gain1/1 -> Sum/2
  Product1/1 -> Product4/1
  M_matrix/1 -> Product1/2
  Product4/1 -> Product3/2
  Constant/1 -> Product4/2
  Product3/1 -> Gain1/1
  [rho] -> Product2/2, Product3/1
  F_matrix/1 -> Product/2
  Product2/1 -> Gain/1

== system UNIFIER_dyn3DOF/UNIFIER OBM1/Aero/WingForces/Right/WingRootForces ==
  flap_defl : Inport
  alpha : Inport  Port=2
  V_node : Inport  Port=3
  DEP_J : Inport  Port=4
  Interpolation Using Prelookup1 : Interpolation_n-D  NumberOfTableDimensions=5  Table=dp_WING_root.CD  ExtrapMethod=Clip  ValidIndexMayReachLast=on  NumSelectionDims=1  InternalRulePriority=Speed  TableDataTypeStr=Inherit: Inherit from 'Table data'
      settings: InputPortMap=u0,u1,u2,u3,u4,u5,u6,u7,u8
  Interpolation Using Prelookup2 : Interpolation_n-D  NumberOfTableDimensions=5  Table=dp_WING_root.CS  ExtrapMethod=Clip  ValidIndexMayReachLast=on  NumSelectionDims=1  InternalRulePriority=Speed  TableDataTypeStr=Inherit: Inherit from 'Table data'
      settings: InputPortMap=u0,u1,u2,u3,u4,u5,u6,u7,u8
  Interpolation Using Prelookup3 : Interpolation_n-D  NumberOfTableDimensions=5  Table=dp_WING_root.CL  ExtrapMethod=Clip  ValidIndexMayReachLast=on  NumSelectionDims=1  InternalRulePriority=Speed  TableDataTypeStr=Inherit: Inherit from 'Table data'
      settings: InputPortMap=u0,u1,u2,u3,u4,u5,u6,u7,u8
  Interpolation Using Prelookup4 : Interpolation_n-D  NumberOfTableDimensions=5  Table=dp_WING_root.CMx  ExtrapMethod=Clip  ValidIndexMayReachLast=on  NumSelectionDims=1  InternalRulePriority=Speed  TableDataTypeStr=Inherit: Inherit from 'Table data'
      settings: InputPortMap=u0,u1,u2,u3,u4,u5,u6,u7,u8
  Interpolation Using Prelookup5 : Interpolation_n-D  NumberOfTableDimensions=5  Table=dp_WING_root.CMy  ExtrapMethod=Clip  ValidIndexMayReachLast=on  NumSelectionDims=1  InternalRulePriority=Speed  TableDataTypeStr=Inherit: Inherit from 'Table data'
      settings: InputPortMap=u0,u1,u2,u3,u4,u5,u6,u7,u8
  Interpolation Using Prelookup6 : Interpolation_n-D  NumberOfTableDimensions=5  Table=dp_WING_root.CMz  ExtrapMethod=Clip  ValidIndexMayReachLast=on  NumSelectionDims=1  InternalRulePriority=Speed  TableDataTypeStr=Inherit: Inherit from 'Table data'
      settings: InputPortMap=u0,u1,u2,u3,u4,u5,u6,u7,u8
  WingRootPreLookup : Subsystem
  CD : Outport
  CS : Outport  Port=2
  CL : Outport  Port=3
  CMx : Outport  Port=4
  CMy : Outport  Port=5
  CMz : Outport  Port=6
  wires:
  Interpolation Using Prelookup6/1 -> CMz/1
  Interpolation Using Prelookup5/1 -> CMy/1
  Interpolation Using Prelookup4/1 -> CMx/1
  Interpolation Using Prelookup3/1 -> CL/1
  Interpolation Using Prelookup2/1 -> CS/1
  alpha/1 -> WingRootPreLookup/2(alpha)
  V_node/1 -> WingRootPreLookup/3(V_node)
  DEP_J/1 -> WingRootPreLookup/4(DEP_J)
  WingRootPreLookup/2(Out2) -> Interpolation Using Prelookup1/2, Interpolation Using Prelookup2/2, Interpolation Using Prelookup3/2, Interpolation Using Prelookup4/2, Interpolation Using Prelookup5/2, Interpolation Using Prelookup6/2
  WingRootPreLookup/6(Out7) -> Interpolation Using Prelookup1/6, Interpolation Using Prelookup2/6, Interpolation Using Prelookup3/6, Interpolation Using Prelookup4/6, Interpolation Using Prelookup5/6, Interpolation Using Prelookup6/6
  Interpolation Using Prelookup1/1 -> CD/1
  WingRootPreLookup/5(Out6) -> Interpolation Using Prelookup2/5, Interpolation Using Prelookup3/5, Interpolation Using Prelookup4/5, Interpolation Using Prelookup5/5, Interpolation Using Prelookup6/5, Interpolation Using Prelookup1/5
  WingRootPreLookup/4(Out4) -> Interpolation Using Prelookup1/4, Interpolation Using Prelookup2/4, Interpolation Using Prelookup3/4, Interpolation Using Prelookup4/4, Interpolation Using Prelookup5/4, Interpolation Using Prelookup6/4
  flap_defl/1 -> WingRootPreLookup/1(flap_defl)
  WingRootPreLookup/7(Out8) -> Interpolation Using Prelookup2/7, Interpolation Using Prelookup3/7, Interpolation Using Prelookup4/7, Interpolation Using Prelookup6/7, Interpolation Using Prelookup5/7, Interpolation Using Prelookup1/7
  WingRootPreLookup/1(Out1) -> Interpolation Using Prelookup1/1, Interpolation Using Prelookup2/1, Interpolation Using Prelookup3/1, Interpolation Using Prelookup4/1, Interpolation Using Prelookup5/1, Interpolation Using Prelookup6/1
  WingRootPreLookup/8(Out9) -> Interpolation Using Prelookup1/8, Interpolation Using Prelookup2/8, Interpolation Using Prelookup3/8, Interpolation Using Prelookup4/8, Interpolation Using Prelookup5/8, Interpolation Using Prelookup6/8
  WingRootPreLookup/3(Out3) -> Interpolation Using Prelookup1/3, Interpolation Using Prelookup2/3, Interpolation Using Prelookup3/3, Interpolation Using Prelookup4/3, Interpolation Using Prelookup5/3, Interpolation Using Prelookup6/3
  WingRootPreLookup/9(Out5) -> Interpolation Using Prelookup1/9, Interpolation Using Prelookup2/9, Interpolation Using Prelookup3/9, Interpolation Using Prelookup4/9, Interpolation Using Prelookup5/9, Interpolation Using Prelookup6/9

== system UNIFIER_dyn3DOF/UNIFIER OBM1/Aero/WingForces/Right/WingTipForces ==
  ail_defl : Inport
  alpha : Inport  Port=2
  V_node : Inport  Port=3
  DEP_J : Inport  Port=4
  Interpolation Using Prelookup1 : Interpolation_n-D  NumberOfTableDimensions=5  Table=dp_WING_tip.CD  ExtrapMethod=Clip  ValidIndexMayReachLast=on  NumSelectionDims=1  InternalRulePriority=Speed  TableDataTypeStr=Inherit: Inherit from 'Table data'
      settings: InputPortMap=u0,u1,u2,u3,u4,u5,u6,u7,u8
  Interpolation Using Prelookup2 : Interpolation_n-D  NumberOfTableDimensions=5  Table=dp_WING_tip.CS  ExtrapMethod=Clip  ValidIndexMayReachLast=on  NumSelectionDims=1  InternalRulePriority=Speed  TableDataTypeStr=Inherit: Inherit from 'Table data'
      settings: InputPortMap=u0,u1,u2,u3,u4,u5,u6,u7,u8
  Interpolation Using Prelookup3 : Interpolation_n-D  NumberOfTableDimensions=5  Table=dp_WING_tip.CL  ExtrapMethod=Clip  ValidIndexMayReachLast=on  NumSelectionDims=1  InternalRulePriority=Speed  TableDataTypeStr=Inherit: Inherit from 'Table data'
      settings: InputPortMap=u0,u1,u2,u3,u4,u5,u6,u7,u8
  Interpolation Using Prelookup4 : Interpolation_n-D  NumberOfTableDimensions=5  Table=dp_WING_tip.CMx  ExtrapMethod=Clip  ValidIndexMayReachLast=on  NumSelectionDims=1  InternalRulePriority=Speed  TableDataTypeStr=Inherit: Inherit from 'Table data'
      settings: InputPortMap=u0,u1,u2,u3,u4,u5,u6,u7,u8
  Interpolation Using Prelookup5 : Interpolation_n-D  NumberOfTableDimensions=5  Table=dp_WING_tip.CMy  ExtrapMethod=Clip  ValidIndexMayReachLast=on  NumSelectionDims=1  InternalRulePriority=Speed  TableDataTypeStr=Inherit: Inherit from 'Table data'
      settings: InputPortMap=u0,u1,u2,u3,u4,u5,u6,u7,u8
  Interpolation Using Prelookup6 : Interpolation_n-D  NumberOfTableDimensions=5  Table=dp_WING_tip.CMz  ExtrapMethod=Clip  ValidIndexMayReachLast=on  NumSelectionDims=1  InternalRulePriority=Speed  TableDataTypeStr=Inherit: Inherit from 'Table data'
      settings: InputPortMap=u0,u1,u2,u3,u4,u5,u6,u7,u8
  WingRootPreLookup : Subsystem
  CD : Outport
  CS : Outport  Port=2
  CL : Outport  Port=3
  CMx : Outport  Port=4
  CMy : Outport  Port=5
  CMz : Outport  Port=6
  wires:
  Interpolation Using Prelookup6/1 -> CMz/1
  Interpolation Using Prelookup5/1 -> CMy/1
  Interpolation Using Prelookup4/1 -> CMx/1
  Interpolation Using Prelookup3/1 -> CL/1
  Interpolation Using Prelookup2/1 -> CS/1
  alpha/1 -> WingRootPreLookup/2(alpha)
  V_node/1 -> WingRootPreLookup/3(V_node)
  DEP_J/1 -> WingRootPreLookup/4(DEP_J)
  WingRootPreLookup/2(Out2) -> Interpolation Using Prelookup1/2, Interpolation Using Prelookup2/2, Interpolation Using Prelookup3/2, Interpolation Using Prelookup4/2, Interpolation Using Prelookup5/2, Interpolation Using Prelookup6/2
  WingRootPreLookup/6(Out7) -> Interpolation Using Prelookup1/6, Interpolation Using Prelookup2/6, Interpolation Using Prelookup3/6, Interpolation Using Prelookup4/6, Interpolation Using Prelookup5/6, Interpolation Using Prelookup6/6
  Interpolation Using Prelookup1/1 -> CD/1
  WingRootPreLookup/5(Out6) -> Interpolation Using Prelookup2/5, Interpolation Using Prelookup3/5, Interpolation Using Prelookup4/5, Interpolation Using Prelookup5/5, Interpolation Using Prelookup6/5, Interpolation Using Prelookup1/5
  WingRootPreLookup/4(Out4) -> Interpolation Using Prelookup1/4, Interpolation Using Prelookup2/4, Interpolation Using Prelookup3/4, Interpolation Using Prelookup4/4, Interpolation Using Prelookup5/4, Interpolation Using Prelookup6/4
  ail_defl/1 -> WingRootPreLookup/1(ail_defl)
  WingRootPreLookup/7(Out8) -> Interpolation Using Prelookup1/7, Interpolation Using Prelookup2/7, Interpolation Using Prelookup3/7, Interpolation Using Prelookup4/7, Interpolation Using Prelookup6/7, Interpolation Using Prelookup5/7
  WingRootPreLookup/1(Out1) -> Interpolation Using Prelookup1/1, Interpolation Using Prelookup2/1, Interpolation Using Prelookup3/1, Interpolation Using Prelookup4/1, Interpolation Using Prelookup5/1, Interpolation Using Prelookup6/1
  WingRootPreLookup/8(Out9) -> Interpolation Using Prelookup1/8, Interpolation Using Prelookup2/8, Interpolation Using Prelookup3/8, Interpolation Using Prelookup4/8, Interpolation Using Prelookup5/8, Interpolation Using Prelookup6/8
  WingRootPreLookup/3(Out3) -> Interpolation Using Prelookup1/3, Interpolation Using Prelookup2/3, Interpolation Using Prelookup3/3, Interpolation Using Prelookup4/3, Interpolation Using Prelookup5/3, Interpolation Using Prelookup6/3
  WingRootPreLookup/9(Out5) -> Interpolation Using Prelookup1/9, Interpolation Using Prelookup2/9, Interpolation Using Prelookup3/9, Interpolation Using Prelookup4/9, Interpolation Using Prelookup5/9, Interpolation Using Prelookup6/9

== system UNIFIER_dyn3DOF/UNIFIER OBM1/Subsystems/DEP1/DEP/Controller ==
  actf : Inport
  Constant3 : Constant  Value=0
  Switch1 : Switch  Criteria=u2 > Threshold  Threshold=0.001  SaturateOnIntegerOverflow=off  InputSameDT=off
  T2rpm : Lookup_n-D  BreakpointsForDimension1=dp_DEP.rpm_lookup.V_vec  BreakpointsForDimension2=dp_DEP.rpm_lookup.T_vec  IndexSearchMethod=Linear search  BeginIndexSearchUsingPreviousIndexResult=on  Table=dp_DEP.rpm_lookup.rpm_gird  ExtrapMethod=Clip  InternalRulePriority=Speed  RndMeth=Simplest
      settings: InputPortMap=u0,u1
  actf2T : Gain  Gain=800
  rpm_cmd : Outport
  wires:
  T2rpm/1 -> Switch1/1
  [V] -> T2rpm/1
  actf/1 -> actf2T/1, Switch1/2
  Switch1/1 -> rpm_cmd/1
  Constant3/1 -> Switch1/3
  actf2T/1 -> T2rpm/2

== system UNIFIER_dyn3DOF/UNIFIER OBM1/Subsystems/DEP1/DEP/Conversion ==
  note: DEP disk inclined 5 degree down
  torque_multiplier : Inport
  Q : Inport  Port=2
  T : Inport  Port=3
  xyz_DEP : Inport  Port=4
  3x3 Cross Product1 : sharedutil/3x3 Cross Product  aMode=aMode
  CG : Constant  Value=xyz_cg
  Cast : DataTypeConversion  OutDataTypeStr=single  SaturateOnIntegerOverflow=off  RndMeth=Floor
  Constant : Constant  Value=0
  Constant1 : Constant  Value=0
  DEP_incidence : Constant  Value=deg2rad(-5)
  Matrix Multiply : Product  Multiplication=Matrix(*)
  Matrix Multiply1 : Product  Multiplication=Matrix(*)
  Minus : Sum  Inputs=+-
  Mux : Mux  Inputs=3
  Mux1 : Mux  Inputs=3
  Mux2 : Mux  Inputs=3
  Product4 : Product
  Rotation Angles to Direction Cosine Matrix : sharedtransform/Rotation Angles to Direction Cosine Matrix  rotationOrder=ZYX  aMode=aMode
  Saturation : Saturate  UpperLimit=inf  LowerLimit=0
  Saturation1 : Saturate  UpperLimit=inf  LowerLimit=0
  Sum2 : Sum  Inputs=++|
  Transpose : Math  Operator=transpose
  F : Outport
  M : Outport  Port=2
  wires:
  Saturation1/1 -> Mux2/1
  T/1 -> Saturation/1
  Transpose/1 -> Matrix Multiply/1, Matrix Multiply1/1
  Q/1 -> Saturation1/1
  Constant/1 -> Mux/2, Mux2/2, Mux2/3, Mux/3
  Sum2/1 -> M/1
  Saturation/1 -> Mux/1
  3x3 Cross Product1/1 -> Sum2/2
  CG/1 -> Cast/1
  xyz_DEP/1 -> Minus/1
  Mux/1 -> Matrix Multiply1/2
  Mux1/1 -> Rotation Angles to Direction Cosine Matrix/1
  Minus/1 -> 3x3 Cross Product1/1
  Constant1/1 -> Mux1/1, Mux1/3
  Cast/1 -> Minus/2
  DEP_incidence/1 -> Mux1/2
  torque_multiplier/1 -> Product4/1
  Mux2/1 -> Matrix Multiply/2
  Matrix Multiply1/1 -> 3x3 Cross Product1/2, F/1
  Product4/1 -> Sum2/1
  Rotation Angles to Direction Cosine Matrix/1 -> Transpose/1
  Matrix Multiply/1 -> Product4/2

== system UNIFIER_dyn3DOF/UNIFIER OBM1/Subsystems/DEP1/DEP/Propeller ==
  n : Inport
  Constant : Constant  Value=eps
  Divide : Product  Inputs=*/
  Gain : Gain  Gain=1.6^5
  Gain2 : Gain  Gain=1.6
  Gain3 : Gain  Gain=1.6^4
  Product{,1..3} (4 alike) : Product
  Propeller data LOOKUP C_Q : Lookup_n-D  NumberOfTableDimensions=1  BreakpointsForDimension1=dp_DEP.J  IndexSearchMethod=Linear search  BeginIndexSearchUsingPreviousIndexResult=on  Table=dp_DEP.C_Q  ExtrapMethod=Clip  UseLastTableValue=on  InternalRulePriority=Speed  RndMeth=Simplest
  Propeller data LOOKUP C_T : Lookup_n-D  NumberOfTableDimensions=1  BreakpointsForDimension1=dp_DEP.J  IndexSearchMethod=Linear search  BeginIndexSearchUsingPreviousIndexResult=on  Table=dp_DEP.C_T  ExtrapMethod=Clip  UseLastTableValue=on  InternalRulePriority=Speed  RndMeth=Simplest
  Saturation : Saturate  UpperLimit=inf  LowerLimit=0
  Saturation1 : Saturate  UpperLimit=2.5  LowerLimit=0.3
  Square : Math  Operator=square
  Sum2 : Sum  Inputs=|++
  J : Outport
  Q : Outport  Port=2
  T : Outport  Port=3
  C_T : Outport  Port=4
  wires:
  n/1 -> Saturation/1
  Saturation1/1 -> Propeller data LOOKUP C_T/1, Propeller data LOOKUP C_Q/1, J/1
  Gain2/1 -> Sum2/1
  Product/1 -> Product1/2
  Square/1 -> Product1/1, Product3/2
  Propeller data LOOKUP C_T/1 -> Product2/2, C_T/1  "C_T"
  Propeller data LOOKUP C_Q/1 -> Product/2  "C_Q"
  Product1/1 -> Gain/1
  Product3/1 -> Gain3/1
  Constant/1 -> Sum2/2
  [V] -> Divide/1
  Divide/1 -> Saturation1/1  "J"
  Gain3/1 -> T/1
  Gain/1 -> Q/1
  Saturation/1 -> Gain2/1, Square/1
  [rho] -> Product/1, Product2/1
  Sum2/1 -> Divide/2
  Product2/1 -> Product3/1

== system UNIFIER_dyn3DOF/UNIFIER OBM1/Aero/WingForces/Left/Subsystem/CrossProduct ==
  r : Inport  Partition=on  PartitionDimension=2  PartitionWidth=1  PartitionOffset=0
  F : Inport  Port=2  Partition=on  PartitionDimension=2  PartitionWidth=1  PartitionOffset=0
  3x3 Cross Product : sharedutil/3x3 Cross Product  aMode=aMode
  CG : Constant  Value=xyz_cg
  Cast : DataTypeConversion  OutDataTypeStr=single  SaturateOnIntegerOverflow=off  RndMeth=Floor
  For Each : ForEach  DisableCoverage=on  SpecifiedNumIters=7
  Minus : Sum  Inputs=+-
  M : Outport  ConcatenationDimension=2
  wires:
  Cast/1 -> Minus/2
  Minus/1 -> 3x3 Cross Product/1
  CG/1 -> Cast/1
  3x3 Cross Product/1 -> M/1
  r/1 -> Minus/1
  F/1 -> 3x3 Cross Product/2

== system UNIFIER_dyn3DOF/UNIFIER OBM1/Aero/WingForces/Left/Subsystem/w2b ==
  alpha : Inport  OutDataTypeStr=single  Partition=on  PartitionDimension=1  PartitionWidth=1  PartitionOffset=0
  Fw : Inport  Port=2  Partition=on  PartitionDimension=2  PartitionWidth=1  PartitionOffset=0
  Cast To Double : DataTypeConversion  OutDataTypeStr=double  SaturateOnIntegerOverflow=off  RndMeth=Floor
  Cast To Single : DataTypeConversion  OutDataTypeStr=single  SaturateOnIntegerOverflow=off  RndMeth=Floor
  Constant : Constant  Value=0  OutDataTypeStr=single
  Demux : Demux  Outputs=3
  Direction Cosine Matrix Body to Wind : aerolibtransform2/Direction Cosine Matrix Body to Wind
  For Each : ForEach  DisableCoverage=on  SpecifiedNumIters=7
  Matrix Multiply : Product  Multiplication=Matrix(*)
  Mux : Mux  Inputs=3
  Mux1 : Mux  Inputs=2
  Transpose : Math  Operator=transpose
  Unary Minus : UnaryMinus
  Unary Minus1 : UnaryMinus
  Fb : Outport  ConcatenationDimension=2
  wires:
  Cast To Double/1 -> Direction Cosine Matrix Body to Wind/1
  Cast To Single/1 -> Matrix Multiply/1
  Constant/1 -> Mux1/2
  Mux1/1 -> Cast To Double/1
  Transpose/1 -> Cast To Single/1
  Direction Cosine Matrix Body to Wind/1 -> Transpose/1
  Demux/3 -> Unary Minus1/1
  Unary Minus1/1 -> Mux/3
  Demux/2 -> Mux/2
  Unary Minus/1 -> Mux/1
  Demux/1 -> Unary Minus/1
  Mux/1 -> Matrix Multiply/2
  Matrix Multiply/1 -> Fb/1
  alpha/1 -> Mux1/1
  Fw/1 -> Demux/1

== system UNIFIER_dyn3DOF/UNIFIER OBM1/Aero/WingForces/Left/WingRootForces/WingRootPreLookup ==
  flap_defl : Inport
  alpha : Inport  Port=2
  V_node : Inport  Port=3
  DEP_J : Inport  Port=4
  Constant8 : Constant  Value=0:4
  Prelookup : PreLookup  BreakpointsData=dp_WING_root.flap_defl  IndexSearchMethod=Linear search  BeginIndexSearchUsingPreviousIndexResult=on  UseLastBreakpoint=on
  Prelookup1 : PreLookup  BreakpointsData=dp_WING_root.alphas  IndexSearchMethod=Linear search  BeginIndexSearchUsingPreviousIndexResult=on  UseLastBreakpoint=on
  Prelookup2 : PreLookup  BreakpointsData=dp_WING_root.V  IndexSearchMethod=Linear search  BeginIndexSearchUsingPreviousIndexResult=on  UseLastBreakpoint=on
  Prelookup3 : PreLookup  BreakpointsData=dp_WING_root.DEP_J  IndexSearchMethod=Linear search  BeginIndexSearchUsingPreviousIndexResult=on  UseLastBreakpoint=on
  Out1 : Outport
  Out2 : Outport  Port=2
  Out3 : Outport  Port=3
  Out4 : Outport  Port=4
  Out6 : Outport  Port=5
  Out7 : Outport  Port=6
  Out8 : Outport  Port=7
  Out9 : Outport  Port=8
  Out5 : Outport  Port=9
  wires:
  Prelookup3/2 -> Out9/1
  Prelookup3/1 -> Out8/1
  Prelookup2/2 -> Out7/1
  Prelookup2/1 -> Out6/1
  DEP_J/1 -> Prelookup3/1
  V_node/1 -> Prelookup2/1
  flap_defl/1 -> Prelookup/1
  Prelookup1/1 -> Out3/1
  alpha/1 -> Prelookup1/1
  Prelookup/2 -> Out2/1
  Prelookup1/2 -> Out4/1
  Constant8/1 -> Out5/1
  Prelookup/1 -> Out1/1

== system UNIFIER_dyn3DOF/UNIFIER OBM1/Aero/WingForces/Left/WingTipForces/WingRootPreLookup ==
  ail_defl : Inport
  alpha : Inport  Port=2
  V_node : Inport  Port=3
  DEP_J : Inport  Port=4
  Constant8 : Constant  Value=0:1
  Prelookup : PreLookup  BreakpointsData=dp_WING_tip.ail_defl  IndexSearchMethod=Linear search  BeginIndexSearchUsingPreviousIndexResult=on  UseLastBreakpoint=on
  Prelookup1 : PreLookup  BreakpointsData=dp_WING_tip.alphas  IndexSearchMethod=Linear search  BeginIndexSearchUsingPreviousIndexResult=on  UseLastBreakpoint=on
  Prelookup2 : PreLookup  BreakpointsData=dp_WING_tip.V  IndexSearchMethod=Linear search  BeginIndexSearchUsingPreviousIndexResult=on  UseLastBreakpoint=on
  Prelookup3 : PreLookup  BreakpointsData=dp_WING_tip.DEP_J  IndexSearchMethod=Linear search  BeginIndexSearchUsingPreviousIndexResult=on  UseLastBreakpoint=on
  Out1 : Outport
  Out2 : Outport  Port=2
  Out3 : Outport  Port=3
  Out4 : Outport  Port=4
  Out6 : Outport  Port=5
  Out7 : Outport  Port=6
  Out8 : Outport  Port=7
  Out9 : Outport  Port=8
  Out5 : Outport  Port=9
  wires:
  Prelookup3/2 -> Out9/1
  Prelookup3/1 -> Out8/1
  Prelookup2/2 -> Out7/1
  Prelookup2/1 -> Out6/1
  DEP_J/1 -> Prelookup3/1
  V_node/1 -> Prelookup2/1
  ail_defl/1 -> Prelookup/1
  Prelookup1/1 -> Out3/1
  alpha/1 -> Prelookup1/1
  Prelookup/2 -> Out2/1
  Prelookup1/2 -> Out4/1
  Constant8/1 -> Out5/1
  Prelookup/1 -> Out1/1
